simulink model "Test_u"  (R2019a)
settings: Solver=VariableStepAuto  StartTime=0.0  StopTime=10.0  RelTol=1e-3
values from neighbouring files (symbols this model uses):
  Stoerung1 = 0.1    [roboMain.m]
libraries: simulink x1
settings Model: Creator=quynh  LastModifiedBy=quynh

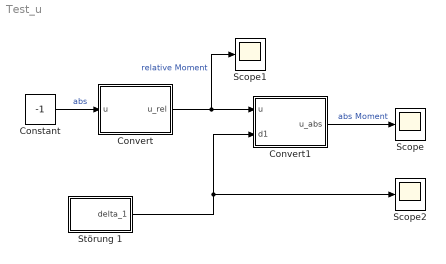
== system Test_u ==
  Constant : Constant  Value=-1
  Convert : MATLAB Function  TreatAsAtomicUnit=on
  Convert1 : MATLAB Function  TreatAsAtomicUnit=on
  Scope : Scope
  Scope1 : Scope
  Scope2 : Scope
  Störung 1 : Subsystem
  wires:
  Convert/1(u_rel) -> Convert1/1(u), Scope1/1  "relative Moment"
  Constant/1 -> Convert/1(u)  "abs"
  Convert1/1(u_abs) -> Scope/1  "abs Moment"
  Störung 1/1("delta_1 ") -> Convert1/2(d1), Scope2/1

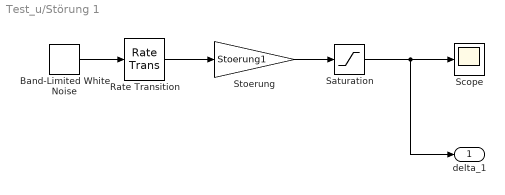
== system Test_u/Störung 1 ==
  Band-Limited White Noise : simulink/Sources/Band-Limited White Noise  Cov=stoerungNoisePower  Ts=0.025  seed=stoerungSeed_1
  Rate Transition : RateTransition
  Saturation : Saturate  UpperLimit=3  LowerLimit=-3
  Scope : Scope
  Stoerung : Gain  Gain=Stoerung1
  "delta_1 " : Outport
  wires:
  Band-Limited White Noise/1 -> Rate Transition/1
  Rate Transition/1 -> Stoerung/1
  Stoerung/1 -> Saturation/1
  Saturation/1 -> "delta_1 "/1, Scope/1

== matlab function Test_u/Convert1 ==
  data: u input; u_abs output; d1 input
function u_abs = fcn(u,d1)    % 
Pmax = 3.56;
umax = 100;
d1 = 0;
Stoerung1 = 0.1;



P = (u+d1)/umax*Pmax; %Leistung eines Motors
M_max = sqrt(abs(P))/9.434;
M = 2*sign(u)*M_max; % Gesamtmoment

u_abs = M;

== matlab function Test_u/Convert ==
  data: u input; u_rel output
function u_rel = fcn(u)    % u ist u_Schlange: absolute u
Pmax = 3.56;


u_rel = 9.434^2/4*u^2*sign(u/2)*100/Pmax;
